simulink model "MotorModel"  (R2015b)
settings: Solver=VariableStepAuto  StartTime=0.0  StopTime=10.0  RelTol=1e-3
undefined symbols (not defined in the file): ArduCopter, b, beta, I_R, init_M, k, l, Motor, throttle_pwm_scalar, Uav
settings Model: Creator=jban039  LastModifiedBy=jeremie

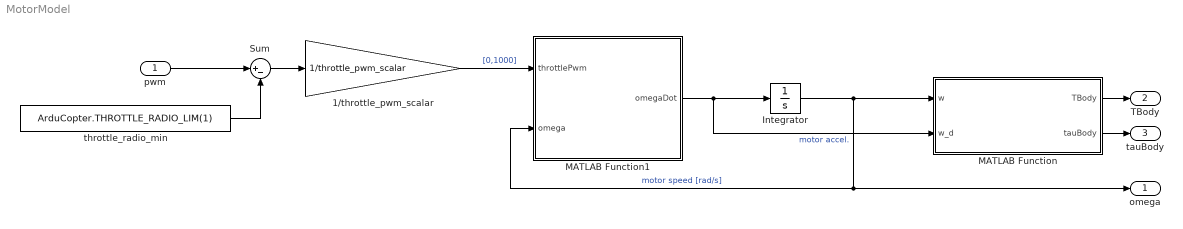
== system MotorModel ==
  pwm : Inport
  1/throttle_pwm_scalar : Gain  Gain=1/throttle_pwm_scalar
  Integrator : Integrator  InitialCondition=init_M
  MATLAB Function : MATLAB Function  TreatAsAtomicUnit=on
  MATLAB Function1 : MATLAB Function  TreatAsAtomicUnit=on
  Sum : Sum  Inputs=|+-
  throttle_radio_min : Constant  Value=ArduCopter.THROTTLE_RADIO_LIM(1)
  omega : Outport
  TBody : Outport  Port=2
  tauBody : Outport  Port=3
  wires:
  MATLAB Function1/1(omegaDot) -> MATLAB Function/2(w_d), Integrator/1  "motor accel."
  MATLAB Function/2(tauBody) -> tauBody/1
  MATLAB Function/1(TBody) -> TBody/1
  Integrator/1 -> MATLAB Function/1(w), omega/1, MATLAB Function1/2(omega)  "motor speed [rad/s]"
  throttle_radio_min/1 -> Sum/2
  Sum/1 -> 1/throttle_pwm_scalar/1
  pwm/1 -> Sum/1
  1/throttle_pwm_scalar/1 -> MATLAB Function1/1(throttlePwm)  "[0,1000]"

== matlab function MotorModel/MATLAB Function ==
  data: w input; TBody output; w_d input; k parameter; b parameter; l parameter; beta parameter; tauBody output; I_R parameter
function [TBody,tauBody] = motorForceTorque(w,w_d, k,b,l,beta,I_R)
%#codegen

% Motor force/torque vectors in motor frame
ind_Mi = (-1).^((1:1:4));
T_Mi = [zeros(2,4); k*(w'.^2)];
tau_Mi = [zeros(2,4); (b*(w'.^2)+I_R(3,3)*w_d').*ind_Mi];

% Initialise matrices to store motor force/torque vectors
T_Bi = zeros(3,4);
tau_Bi = zeros(3,4);

% Calculate forces and moments from each motor in the body frame
for i=1:4
	% Matrix to calculate moments in body frame due to rotor thrust
 	R_F_B = [ 0,              0,              l*sin(beta(i)) ;
              0,              0,             -l*cos(beta(i)) ;
             -l*sin(beta(i)), l*cos(beta(i)), 0             ];

	% Motor force/torque vectors in body frame
	T_Bi(:,i) = T_Mi(:,i);
	tau_Bi(:,i) = tau_Mi(:,i)+R_F_B*T_Mi(:,i);
end

% Total force/torque in body frame
TBody = sum(T_Bi,2);
tauBody = sum(tau_Bi,2);

end

== matlab function MotorModel/MATLAB Function1 ==
  data: throttlePwm input; omegaDot output double size=4; omega input; Motor parameter; Uav parameter
function omegaDot = motorAcceleration(throttlePwm, omega, Motor, Uav)
%#codegen

% applied motor voltages
voltage = throttlePwm * Uav.NOMINAL_BATTERY_VOLTAGE / 1000;

% motor current, ignoring inductance
current = (voltage - Motor.K_E*omega) / Motor.R;

netTorque = (Motor.K_T * current) - (Motor.B * omega.^2);

omegaDot = netTorque / Motor.I_R(3,3);  % motor angular acceleration
